simulink model "hw2simulink"  (R2024b)
settings: Solver=VariableStepAuto  StartTime=0.0  StopTime=10.0  RelTol=1e-3
settings Model: Creator=eitherwoods  LastModifiedBy=eitherwoods

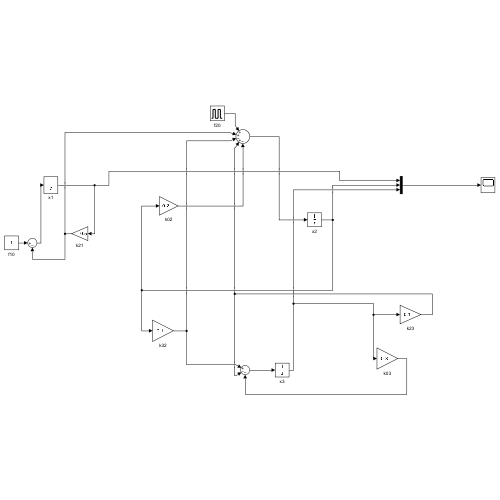
[thumbnail: Simulink's stored preview of the top-level diagram]
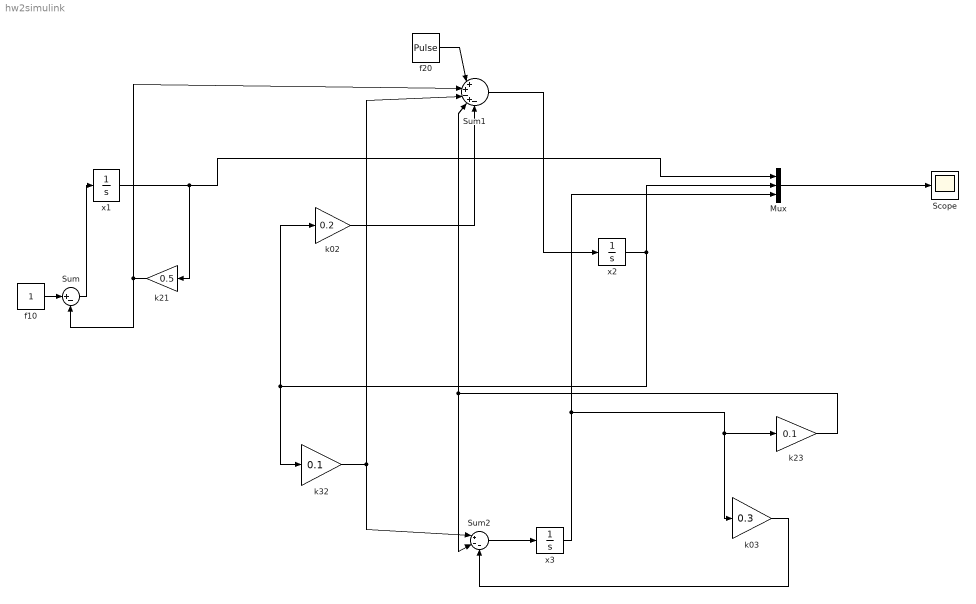
== system hw2simulink ==
  Mux : Mux  Inputs=3
  Scope : Scope
  Sum : Sum  Inputs=|+-
  Sum1 : Sum  Inputs=|++-+-
  Sum2 : Sum  Inputs=|+--
  f10 : Constant
  f20 : DiscretePulseGenerator  PulseType=Time based  Amplitude=10000  Period=10000  PulseWidth=0.001
  k02 : Gain  Gain=0.2
  k03 : Gain  Gain=0.3
  k21 : Gain  Gain=0.5
  k23 : Gain  Gain=0.1
  k32 : Gain  Gain=0.1
  x1 : Integrator
  x2 : Integrator
  x3 : Integrator
  wires:
  x1/1 -> k21/1, Mux/1
  Sum/1 -> x1/1
  k21/1 -> Sum1/2, Sum/2
  f10/1 -> Sum/1
  Mux/1 -> Scope/1
  x3/1 -> Mux/3, k03/1, k23/1
  Sum1/1 -> x2/1
  f20/1 -> Sum1/1
  k23/1 -> Sum2/2, Sum1/4
  k32/1 -> Sum1/3, Sum2/1
  x2/1 -> Mux/2, k02/1, k32/1
  k02/1 -> Sum1/5
  Sum2/1 -> x3/1
  k03/1 -> Sum2/3
